simulink model "simlab14"  (R2022b)
settings: Solver=VariableStepAuto  StartTime=0.0  StopTime=t_simulation  MaxStep=0.1  RelTol=1e-3
values from neighbouring files (symbols this model uses):
  Final_value = 1.5    [laby14.m]
  K = 5    [laby14.m]
  T = 9    [laby14.m]
  t0 = 2    [laby14.m]
  t_start = 10    [laby14.m]
  Value_0 = 0    [laby14.m]
settings Model: Creator=huber  LastModifiedBy=huber
settings DataIOCC: ReturnWorkspaceOutputs=off

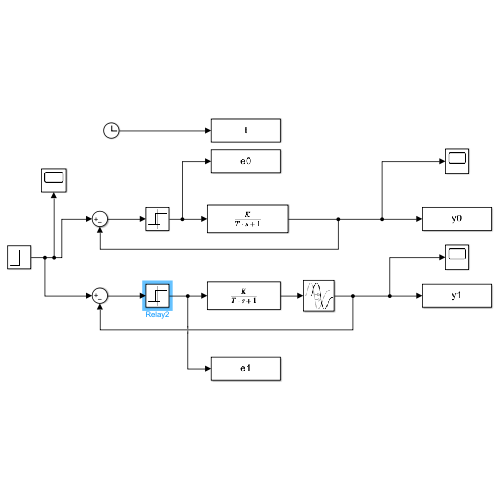
[thumbnail: Simulink's stored preview of the top-level diagram]
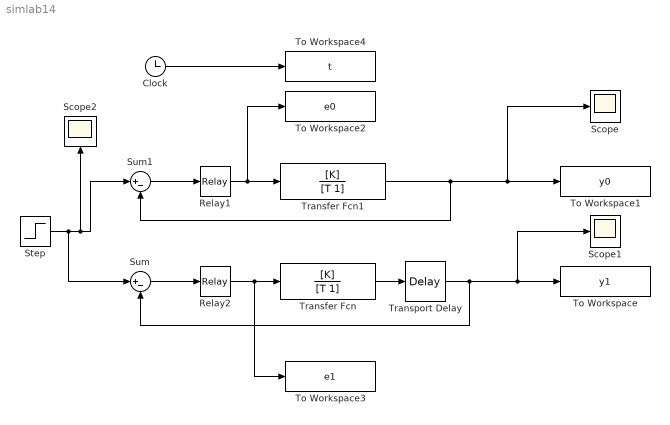
== system simlab14 ==
  Clock : Clock
  Relay1 : Relay  OnSwitchValue=max  OffSwitchValue=min
  Relay2 : Relay  OnSwitchValue=max  OffSwitchValue=min
  Scope : Scope
  Scope1 : Scope
  Scope2 : Scope
  Step : Step  Time=t_start  Before=Value_0  After=Final_value  SampleTime=0
  Sum : Sum  Inputs=|+-
  Sum1 : Sum  Inputs=|+-
  To Workspace : ToWorkspace  VariableName=y1  SampleTime=-1
  To Workspace1 : ToWorkspace  VariableName=y0  SampleTime=-1
  To Workspace2 : ToWorkspace  VariableName=e0  SampleTime=-1
  To Workspace3 : ToWorkspace  VariableName=e1  SampleTime=-1
  To Workspace4 : ToWorkspace  VariableName=t  SampleTime=-1
  Transfer Fcn : TransferFcn  Numerator=[K]  Denominator=[T 1]
  Transfer Fcn1 : TransferFcn  Numerator=[K]  Denominator=[T 1]
  Transport Delay : TransportDelay  DelayTime=t0
  wires:
  Step/1 -> Sum/1, Scope2/1, Sum1/1
  Transfer Fcn/1 -> Transport Delay/1
  Transport Delay/1 -> Scope1/1, To Workspace/1, Sum/2
  Sum1/1 -> Relay1/1
  Relay1/1 -> To Workspace2/1, Transfer Fcn1/1
  Transfer Fcn1/1 -> Scope/1, To Workspace1/1, Sum1/2
  Clock/1 -> To Workspace4/1
  Sum/1 -> Relay2/1
  Relay2/1 -> To Workspace3/1, Transfer Fcn/1
